simulink model "trajectory_planning1"  (R2019a)
settings: Solver=FixedStepAuto  StartTime=0.0  StopTime=5  FixedStep=1  RelTol=1e-3
libraries: simulink x1
settings Model: Creator=vongu  LastModifiedBy=DongDung
settings DataIOCC: ReturnWorkspaceOutputs=off
settings DebuggingCC: PregeneratedLibrarySubsystemCodeDiagnostic=none  ArithmeticOperatorsInVariantConditions=warning
settings SFSimCC: SimUseLocalCustomCode=off
settings RTWCC: RTWUseLocalCustomCode=off

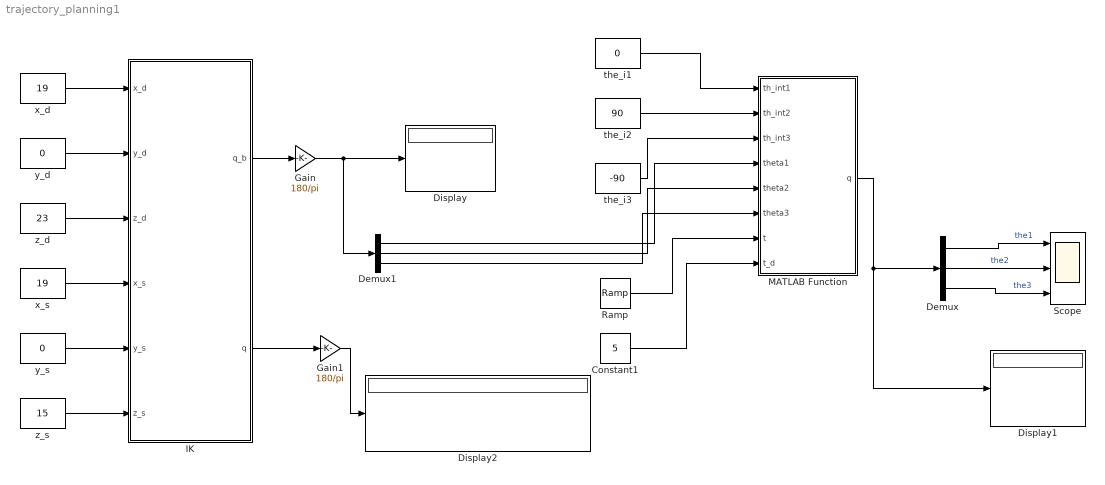
== system trajectory_planning1 ==
  Constant1 : Constant  Value=5  SampleTime=-1
  Demux : Demux  Outputs=3
  Demux1 : Demux  Outputs=3
  Display : Display
  Display1 : Display
  Display2 : Display
  Gain : Gain  Gain=180/pi
  Gain1 : Gain  Gain=180/pi
  IK : MATLAB Function  TreatAsAtomicUnit=on
  MATLAB Function : MATLAB Function  TreatAsAtomicUnit=on
  Ramp : simulink/Sources/Ramp  slope=1  start=0  InitialOutput=0
  Scope : Scope  NumInputPorts=3
  the_i1 : Constant  Value=0  SampleTime=-1
  the_i2 : Constant  Value=90  SampleTime=-1
  the_i3 : Constant  Value=-90  SampleTime=-1
  x_d : Constant  Value=19  SampleTime=-1
  x_s : Constant  Value=19  SampleTime=-1
  y_d : Constant  Value=0  SampleTime=-1
  y_s : Constant  Value=0  SampleTime=-1
  z_d : Constant  Value=23  SampleTime=-1
  z_s : Constant  Value=15  SampleTime=-1
  wires:
  Gain/1 -> Demux1/1, Display/1
  IK/1(q_b) -> Gain/1
  x_s/1 -> IK/4(x_s)
  y_s/1 -> IK/5(y_s)
  z_s/1 -> IK/6(z_s)
  z_d/1 -> IK/3(z_d)
  y_d/1 -> IK/2(y_d)
  x_d/1 -> IK/1(x_d)
  Demux1/3 -> MATLAB Function/6(theta3)
  Ramp/1 -> MATLAB Function/7(t)
  the_i3/1 -> MATLAB Function/3(th_int3)
  Demux/2 -> Scope/2  "the2"
  the_i2/1 -> MATLAB Function/2(th_int2)
  Demux1/1 -> MATLAB Function/4(theta1)
  Demux/3 -> Scope/3  "the3"
  MATLAB Function/1(q) -> Demux/1, Display1/1
  Demux/1 -> Scope/1  "the1"
  the_i1/1 -> MATLAB Function/1(th_int1)
  Demux1/2 -> MATLAB Function/5(theta2)
  Constant1/1 -> MATLAB Function/8(t_d)
  Gain1/1 -> Display2/1
  IK/2(q) -> Gain1/1

== matlab function trajectory_planning1/MATLAB Function ==
  data: th_int1 input; th_int2 input; th_int3 input; q output; theta1 input; theta2 input; theta3 input; t input; t_d input
function q  = fcn(th_int1, th_int2, th_int3, theta1, theta2, theta3, t, t_d )
a1 = th_int1;
b1 = 0;
c1=  3*(theta1-th_int1)/ t_d^2;
d1= -2*(theta1-th_int1)/ t_d^3;
q1 = a1 + b1 * t + c1 * t^2 + d1 * t^3;

a2 = th_int2;
b2 = 0;
c2=  3*(theta2-th_int2)/ t_d^2;
d2= -2*(theta2-th_int2)/ t_d^3;
q2 = a2 + b2 * t + c2 * t^2 + d2 * t^3;

a3 = th_int3;
b3 = 0;
c3=  3*(theta3-th_int3)/ t_d^2;
d3= -2*(theta3-th_int3)/ t_d^3;
q3 = a3 + b3 * t + c3 * t^2 + d3 * t^3;

if t>t_d
  t_d = 0;
end

q=[q1,q2,q3];

== matlab function trajectory_planning1/IK ==
  data: x_d input; y_d input; z_d input; x_s input; y_s input; q_b output; z_s input; q output
function [q_b, q]   = fcn( x_d, y_d, z_d, x_s, y_s, z_s)
L1 = 11; L2 = 23; L3 = 19; d = 4;
q_s= zeros(4,3);
q_b = zeros(1,3);
q1_d = atan2(y_d,x_d);
q11_d = - (pi - q1_d);
costhe3_d = (x_d^2+y_d^2+z_d^2-L2^2-L3^2)/(2*L2*L3);
q31_d = atan2(-sqrt(1-costhe3_d^2),costhe3_d);
q32_d = atan2(sqrt(1-costhe3_d^2),costhe3_d);
q33_d = q31_d;
q34_d = q32_d;
q21_d = atan2(z_d,sqrt(x_d^2+y_d^2))-atan2(L3*sin(q31_d),L2+L3*cos(q31_d));
q22_d = atan2(z_d,sqrt(x_d^2+y_d^2))-atan2(L3*sin(q32_d),L2+L3*cos(q32_d));
q23_d = pi - q22_d;
q24_d = pi - q21_d;

 
q1_s = atan2(y_s,x_s);
q11_s = - (pi - q1_s);
costhe3_s = (x_s^2+y_s^2+z_s^2-L2^2-L3^2)/(2*L2*L3);
q31_s = atan2(-sqrt(1-costhe3_s^2),costhe3_s);
q32_s = atan2(sqrt(1-costhe3_s^2),costhe3_s);
q33_s = q31_s;
q34_s = q32_s;
q21_s = atan2(z_s,sqrt(x_s^2+y_s^2))-atan2(L3*sin(q31_s),L2+L3*cos(q31_s));
q22_s = atan2(z_s,sqrt(x_s^2+y_s^2))-atan2(L3*sin(q32_s),L2+L3*cos(q32_s));
q23_s = pi-q22_s;
q24_s = pi - q21_s;



e1 = (q1_s - q1_d )^2 + (q21_s - q21_d)^2 + (q31_s - q31_d )^2;
e2 = (q1_s - q1_d )^2 + (q22_s - q22_d)^2 + (q32_s - q32_d )^2;
e3 = (q11_s - q11_d )^2 + (q23_s - q23_d)^2 + (q33_s - q33_d )^2;
e4 = (q11_s - q11_d )^2 + (q24_s - q24_d)^2 + (q34_s - q34_d )^2;
e = [e1 e2 e3 e4 ];
min_e = min(e);

  if e1 == min_e
    q_b1 = q1_s;
    q_b2 = q21_s;
    q_b3 = q31_s;
  elseif e2 == min_e
    q_b1 = q1_s;
    q_b2 = q22_s;
    q_b3 = q32_s;
  elseif e3 == min_e
    q_b1 = q11_s;
    q_b2 = q23_s;
    q_b3 = q33_s;
  else 
    q_b1 = q11_s;
    q_b2 = q24_s;
    q_b3 = q34_s;
  end
  
q=[q1_s q21_s q31_s;q1_s q22_s q32_s ;q11_s q23_s q33_s ;q11_s q24_s q34_s];


q_b = [q_b1 q_b2 q_b3];
